simulink model "Version14_2019"  (R2021b)
settings: Solver=VariableStepAuto  StartTime=0.0  StopTime=1320  RelTol=1e-3
values from neighbouring files (symbols this model uses):
  b_clamp = 15    [Version14.m]
  b_zero = 3    [Version14.m]
  dt1 = t1(2) - t1(1)    [Version14.m]
  dt2 = t2(2) - t2(1)    [Version14.m]
  Kb = x(4)    [Version14.m]
  P_future = x(2)    [Version14.m]
  P_now = x(1)    [Version14.m]
  P_offset = x(3)    [Version14.m]
libraries: simulink x1
settings Model: Creator=DC  LastModifiedBy=DC
settings SolverCC: ZeroCrossAlgorithm=Adaptive  AlgebraicLoopSolver=TrustRegion
settings DebuggingCC: MaskedZcDiagnostic=none  IgnoredZcDiagnostic=none
settings SFSimCC: CustomCodeUndefinedFunction=UseInterfaceOnly

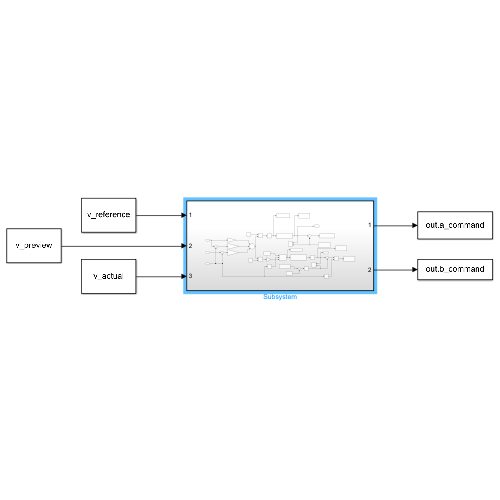
[thumbnail: Simulink's stored preview of the top-level diagram]
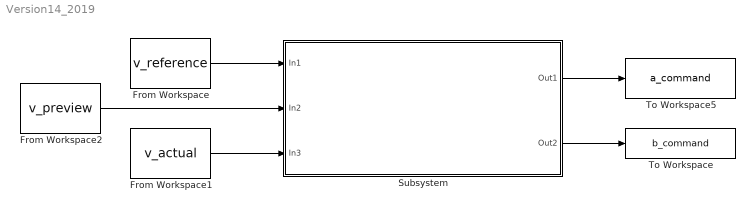
== system Version14_2019 ==
  From Workspace : FromWorkspace  VariableName=v_reference  SampleTime=dt1
  From Workspace1 : FromWorkspace  VariableName=v_actual  SampleTime=dt2
  From Workspace2 : FromWorkspace  VariableName=v_preview  SampleTime=dt1
  Subsystem : Subsystem
  To Workspace : ToWorkspace  VariableName=b_command  SaveFormat=Timeseries  SampleTime=-1
  To Workspace5 : ToWorkspace  VariableName=a_command  SaveFormat=Timeseries  SampleTime=-1
  wires:
  From Workspace/1 -> Subsystem/1(In1)
  From Workspace1/1 -> Subsystem/3(In3)
  Subsystem/1(Out1) -> To Workspace5/1
  Subsystem/2(Out2) -> To Workspace/1
  From Workspace2/1 -> Subsystem/2(In2)

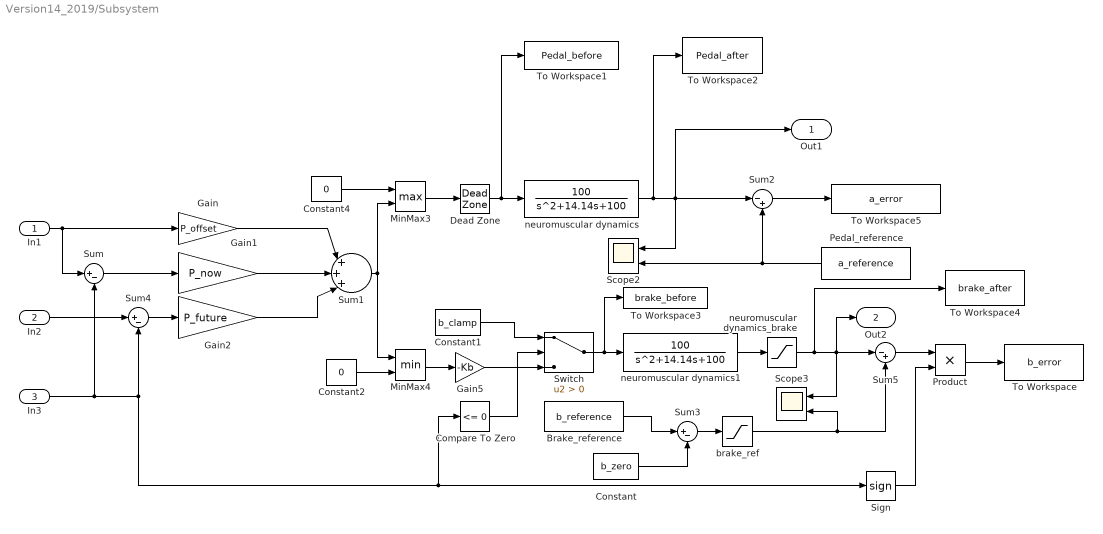
== system Version14_2019/Subsystem ==
  In1 : Inport
  In2 : Inport  Port=2
  In3 : Inport  Port=3
  Brake_reference : FromWorkspace  VariableName=b_reference  SampleTime=dt2
  Compare To Zero : simulink/Logic and Bit Operations/Compare To Zero  relop=<=  OutDataTypeStr=boolean
  Constant : Constant  Value=b_zero
  Constant1 : Constant  Value=b_clamp
  Constant2 : Constant  Value=0
  Constant4 : Constant  Value=0
  Dead Zone : DeadZone  LowerValue=0  UpperValue=a_threshold  SaturateOnIntegerOverflow=on
  Gain : Gain  Gain=P_offset
  Gain1 : Gain  Gain=P_now
  Gain2 : Gain  Gain=P_future
  Gain5 : Gain  Gain=-Kb
  MinMax3 : MinMax  Function=max  Inputs=2
  MinMax4 : MinMax  Inputs=2
  Pedal_reference : FromWorkspace  VariableName=a_reference  SampleTime=dt2
  Product : Product
  Scope2 : Scope  NumInputPorts=2
  Scope3 : Scope  NumInputPorts=2
  Sign : Signum
  Sum : Sum  Inputs=|+-
  Sum1 : Sum  Inputs=|+++|
  Sum2 : Sum  Inputs=|-+
  Sum3 : Sum  Inputs=|+-
  Sum4 : Sum  Inputs=|+-
  Sum5 : Sum  Inputs=|-+
  Switch : Switch  Criteria=u2 > Threshold
  To Workspace : ToWorkspace  VariableName=b_error  SaveFormat=Timeseries  SampleTime=-1
  To Workspace1 : ToWorkspace  VariableName=Pedal_before  SaveFormat=Timeseries  SampleTime=-1
  To Workspace2 : ToWorkspace  VariableName=Pedal_after  SaveFormat=Timeseries  SampleTime=-1
  To Workspace3 : ToWorkspace  VariableName=brake_before  SaveFormat=Timeseries  SampleTime=-1
  To Workspace4 : ToWorkspace  VariableName=brake_after  SaveFormat=Timeseries  SampleTime=-1
  To Workspace5 : ToWorkspace  VariableName=a_error  SaveFormat=Timeseries  SampleTime=-1
  brake_ref : Saturate  UpperLimit=100  LowerLimit=0
  neuromuscular dynamics : TransferFcn  Numerator=[100]  Denominator=[1 14.14 100]
  neuromuscular dynamics1 : TransferFcn  Numerator=[100]  Denominator=[1 14.14 100]
  neuromuscular dynamics_brake : Saturate  UpperLimit=100  LowerLimit=0
  Out1 : Outport
  Out2 : Outport  Port=2
  wires:
  Sum1/1 -> MinMax4/1, MinMax3/2
  Sum/1 -> Gain1/1
  In1/1 -> Sum/1, Gain/1
  MinMax3/1 -> Dead Zone/1
  Constant4/1 -> MinMax3/1
  Gain1/1 -> Sum1/2
  MinMax4/1 -> Gain5/1
  Gain/1 -> Sum1/1
  Sign/1 -> Product/2
  Pedal_reference/1 -> Scope2/2, Sum2/2
  Sum2/1 -> To Workspace5/1
  Product/1 -> To Workspace/1
  Brake_reference/1 -> Sum3/1
  Constant/1 -> Sum3/2
  Sum3/1 -> brake_ref/1
  Sum5/1 -> Product/1
  In2/1 -> Sum4/1
  In3/1 -> Sum/2, Sum4/2, Compare To Zero/1, Sign/1
  Gain2/1 -> Sum1/3
  neuromuscular dynamics/1 -> Sum2/1, Scope2/1, Out1/1, To Workspace2/1
  Compare To Zero/1 -> Switch/2
  Constant1/1 -> Switch/1
  Gain5/1 -> Switch/3
  Dead Zone/1 -> To Workspace1/1, neuromuscular dynamics/1
  Sum4/1 -> Gain2/1
  Constant2/1 -> MinMax4/2
  Switch/1 -> To Workspace3/1, neuromuscular dynamics1/1
  neuromuscular dynamics1/1 -> neuromuscular dynamics_brake/1
  brake_ref/1 -> Scope3/2, Sum5/2
  neuromuscular dynamics_brake/1 -> To Workspace4/1, Scope3/1, Out2/1, Sum5/1
